simulink model "sfcndemo_sfunmem"  (Simulink 7.6)
settings: Solver=FixedStepDiscrete  StartTime=0.0  StopTime=.5  RelTol=1e-3
Description:
  | One step delay and hold "memory" C-MEX S-function
settings Model: Creator=The MathWorks Inc.  ExtModeTrigMode=oneshot  ExtModeArmWhenConnect=off  ExtModeAutoUpdateStatusClock=off
settings DataIOCC: LimitDataPoints=off
settings OptimizationCC: BooleanDataType=off  InitFltsAndDblsToZero=on
settings DebuggingCC: SaveWithParameterizedLinksMsg=none  SignalResolutionControl=TryResolveAllWithWarning  SolverPrmCheckMsg=none  MultiTaskDSMMsg=warning  MultiTaskCondExecSysMsg=none
settings HardwareCC: TargetUnknown=on
settings RTWCC: IncludeERTFirstTime=on
settings CodeAppCC: CustomSymbolStrFcn=$F$N$M
settings GRTTargetCC: TargetFcnLib=ansi_tfl_tmw.mat

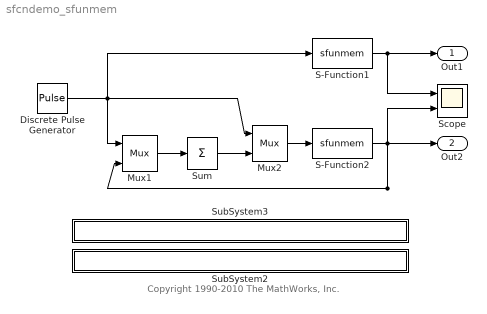
== system sfcndemo_sfunmem ==
  note: Copyright 1990-2010 The MathWorks, Inc.
  Discrete Pulse Generator : DiscretePulseGenerator  Period=20  PulseWidth=10  SampleTime=.01
  Mux1 : Mux  Inputs=2
  Mux2 : Mux  Inputs=2
  S-Function1 : S-Function  FunctionName=sfunmem  EnableBusSupport=off
      mask Type: S-function: sfunmem
      mask Description: This is a S-function block which has one integration-step delay and hold "memory" function.
  S-Function2 : S-Function  FunctionName=sfunmem  EnableBusSupport=off
      mask Type: S-function: sfunmem
      mask Description: This is a S-function block which has one integration-step delay and hold "memory" function.
  Scope : Scope  NumInputPorts=2
      settings: TimeRange=0.5  YMin=0~0  YMax=1~60
  SubSystem2 : Subsystem  mask{filename=sfunmem.tlc}
      mask init:
      | x=sfundemo_maskdisp;
      settings: AttributesFormatString=\n  OpenFcn=sfundemo_openfcn
      mask Display: disp(x);
  SubSystem3 : Subsystem  mask{filename=sfunmem.c}
      mask init:
      | x=sfundemo_maskdisp;
      settings: AttributesFormatString=\n  OpenFcn=sfundemo_openfcn
      mask Display: disp(x);
  Sum : Sum  Inputs=+  SaturateOnIntegerOverflow=on  InputSameDT=on  OutDataTypeStr=Inherit: Same as first input
  Out1 : Outport
  Out2 : Outport  Port=2
  wires:
  Mux1/1 -> Sum/1
  S-Function2/1 -> Mux1/2, Scope/2, Out2/1
  Sum/1 -> Mux2/2
  Mux2/1 -> S-Function2/1
  Discrete Pulse Generator/1 -> S-Function1/1, Mux1/1, Mux2/1
  S-Function1/1 -> Out1/1, Scope/1

== system sfcndemo_sfunmem/SubSystem2 ==

== system sfcndemo_sfunmem/SubSystem3 ==
